simulink model "TPUnSimu"  (R2026a)
settings: Solver=VariableStepAuto

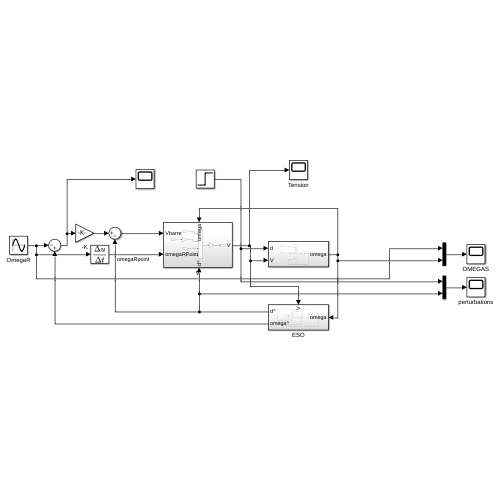
[thumbnail: Simulink's stored preview of the top-level diagram]
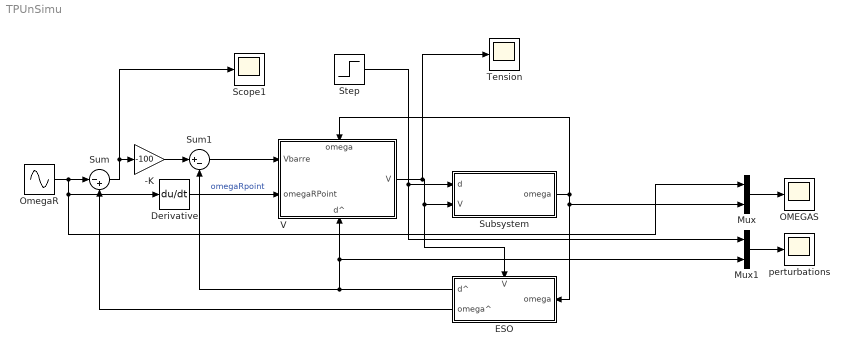
== system TPUnSimu ==
  -K : Gain  Gain=-100
  Derivative : Derivative
  ESO : Subsystem
      settings: PortSchema="{\"entries\":[{\"content\":{\"sides\":[{\"content\":{\"connectorIds\":[\"In1\"]},\"type\":\"ConnectorPlacement.EquallySpacedRectSide\",\"uuid\":\"e1c274ad-ba20-48aa-bf77-d813922b9d8c\"},{\"content\":{\"connectorIds\":[\"Out1\",\"Out2\"],\"side\":\"RIGHT\"},\"type\":\"ConnectorPlacement.EquallySpacedRectSide\",\"uuid\":\"e0452d8d-59d0-4149-8f5d-8992181ff20f\"},{\"content\":{\"connectorIds\":[\"In2\"],\"side\":\"TOP\"},\"type\":\"ConnectorPlacement.EquallySpacedRectSide\",\"uuid\":\"2555fc7c-6481-4291-bd13-a8877dfa9dc8\"}]},\"type\":\"ConnectorPlacement.EquallySpacedConnector\",\"uuid\":\"299a756b-03db-4de2-a07a-503eb175a86e\"}],\"packageUris\":[\"http://schema.mathworks.com/mf0/Connector/R2020b\"],\"version\":\"1.0\"}"
  Mux : Mux  Inputs=2
  Mux1 : Mux  Inputs=2
  OMEGAS : Scope
      settings: ActiveDisplayYMinimum=-0.75962130298935693  ActiveDisplayYMaximum=6.8365917269042145
  OmegaR : Sin  Amplitude=2  Bias=4  Frequency=0.5  SampleTime=0
  Scope1 : Scope
      settings: ActiveDisplayYMinimum=-4.5009372397014058  ActiveDisplayYMaximum=0.5084351573126491
  Step : Step  Time=3  FinalValue=2  SampleTime=0
  Subsystem : Subsystem
  Sum : Sum  Inputs=|-+
  Sum1 : Sum  Inputs=|+-
  Tension : Scope
      settings: ActiveDisplayYMinimum=-0.75075041638227336  ActiveDisplayYMaximum=6.7567537474404622  DataLoggingVariableName=ScopeData3
  V : Subsystem
      settings: PortSchema="{\"entries\":[{\"content\":{\"sides\":[{\"content\":{\"connectorIds\":[\"In1\",\"In2\"]},\"type\":\"ConnectorPlacement.EquallySpacedRectSide\",\"uuid\":\"3806cb88-ac27-4e54-9602-5c269981dd4a\"},{\"content\":{\"connectorIds\":[\"Out1\"],\"side\":\"RIGHT\"},\"type\":\"ConnectorPlacement.EquallySpacedRectSide\",\"uuid\":\"4ee9a9f2-7c78-4ee8-8e7a-01ce00e7f290\"},{\"content\":{\"connectorIds\":[\"In3\"],\"side\":\"TOP\"},\"type\":\"ConnectorPlacement.EquallySpacedRectSide\",\"uuid\":\"e264f9c5-56fc-47fc-809a-fa74c803b869\"},{\"content\":{\"connectorIds\":[\"In4\"],\"side\":\"BOTTOM\"},\"type\":\"ConnectorPlacement.EquallySpacedRectSide\",\"uuid\":\"4158efb2-b17f-4939-9c93-ac5329091cca\"}]},\"type\":\"ConnectorPlacement.EquallySpacedConnector\",\"uuid\":\"47b4022f-b71e-4683-9257-d4ec3ed1dae1\"}],\"packageUris\":[\"http://schema.mathworks.com/mf0/Connector/R2020b\"],\"version\":\"1.0\"}"
  perturbations : Scope
      settings: ActiveDisplayYMinimum=-0.250000003080552  ActiveDisplayYMaximum=2.2500000277249681  DataLoggingVariableName=ScopeData2
  wires:
  Subsystem/1(omega) -> Mux/2, ESO/1(omega), V/3(omega)
  V/1(V) -> Tension/1, ESO/2(V), Subsystem/2(V)
  OmegaR/1 -> Mux/1, Derivative/1, Sum/1
  ESO/2(omega^) -> Sum/2
  Derivative/1 -> V/2(omegaRPoint)  "omegaRpoint"
  Sum/1 -> Scope1/1, -K/1
  -K/1 -> Sum1/1
  Sum1/1 -> V/1(Vbarre)
  Mux/1 -> OMEGAS/1
  Mux1/1 -> perturbations/1
  Step/1 -> Mux1/1, Subsystem/1(d)
  ESO/1(d^) -> Mux1/2, V/4(d^), Sum1/2

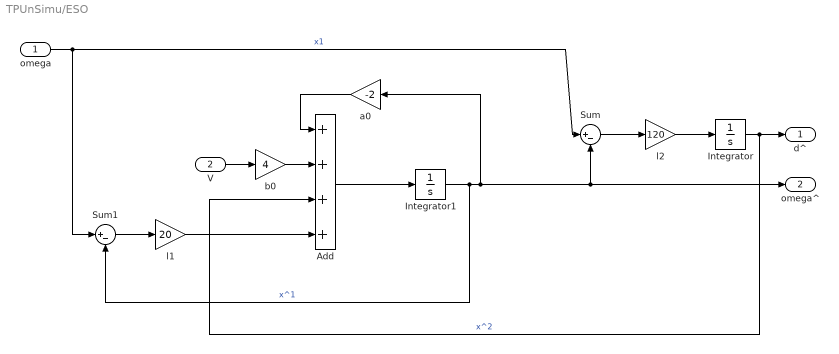
== system TPUnSimu/ESO ==
  omega : Inport
  V : Inport  Port=2
  Add : Sum  Inputs=++++
  Integrator : Integrator
  Integrator1 : Integrator
  Sum : Sum  Inputs=|+-
  Sum1 : Sum  Inputs=|+-
  a0 : Gain  Gain=-2
  b0 : Gain  Gain=4
  l1 : Gain  Gain=20
  l2 : Gain  Gain=120
  d^ : Outport
  omega^ : Outport  Port=2
  wires:
  Integrator/1 -> Add/3, d^/1  "x^2"
  l2/1 -> Integrator/1
  Sum/1 -> l2/1
  omega/1 -> Sum/1, Sum1/1  "x1"
  Integrator1/1 -> omega^/1, Sum/2, a0/1, Sum1/2  "x^1"
  Add/1 -> Integrator1/1
  a0/1 -> Add/1
  V/1 -> b0/1
  b0/1 -> Add/2
  l1/1 -> Add/4
  Sum1/1 -> l1/1

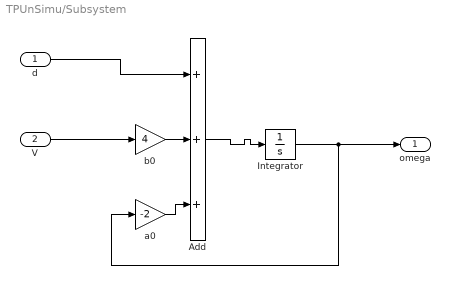
== system TPUnSimu/Subsystem ==
  d : Inport
  V : Inport  Port=2
  Add : Sum  Inputs=+++
  Integrator : Integrator
  a0 : Gain  Gain=-2
  b0 : Gain  Gain=4
  omega : Outport
  wires:
  d/1 -> Add/1
  a0/1 -> Add/3
  Integrator/1 -> a0/1, omega/1
  Add/1 -> Integrator/1
  V/1 -> b0/1
  b0/1 -> Add/2

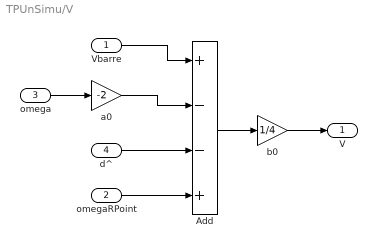
== system TPUnSimu/V ==
  Vbarre : Inport
  omegaRPoint : Inport  Port=2
  omega : Inport  Port=3
  d^ : Inport  Port=4
  Add : Sum  Inputs=+--+
  a0 : Gain  Gain=-2
  b0 : Gain  Gain=1/4
  V : Outport
  wires:
  b0/1 -> V/1
  omegaRPoint/1 -> Add/4
  d^/1 -> Add/3
  a0/1 -> Add/2
  Add/1 -> b0/1
  Vbarre/1 -> Add/1
  omega/1 -> a0/1
